simulink model "SpaceRendezvousAndDockingExample"  (R2025a)
settings: Solver=ode45  StartTime=0.0  StopTime=endTime  RelTol=1e-10  AbsTol=1e-10
PreLoadFcn:
  | % Variables to allow model to run without example script
  | primaryAlignmentVector = [1;0;0];
  | secondaryAlignmentVector = [0;0;1];
  | endTime = 100000;
  | epochYear = 2022;
  | epochMonth = 8;
  | epochDay = 6;
  | epochHour = 0;
  | epochMinute = 0;
  | epochSecond = 0;
  | initialApproachClosingRate = 0.3;
  | finalApproachClosingRate1 = 0.3;
  | finalApproachClosingRate2 = 0.03;
  | primaryConstraintVectorTarget = [1;0;0];
  | secondaryConstraintVectorTarget= [0;0;1];
  | collisionAvoidanceZOffset = 20;
  | transpositionFinalPosition = [20;0;0];
  | m0 = 1000;
  | mDot = 7500;
  | ve = 3924;
  | initialTargetSemimajorAxis = 8000000;
  | initialTargetEccentricity = 0.0005;
  | initialTargetInclination = 30;
  | initialTargetRightAscensionofAscendingNode = 60;
  | initialTargetArgumentOfPeriapsis = 120;
  | initialTargetTrueAnomaly = 310;
  | targetAttitude = [1 0 0 0];
  | initialChaserSemimajorAxis = 7500000;
  | initialChaserEccentricity = 0.001;
  | initialChaserInclination = 30.1;
  | initialChaserRightAscensionofAscendingNode = 60.1;
  | initialChaserArgumentOfPeriapsis = 120;
  | initialChaserTrueAnomaly = 30;
  | burnDirection1 = [-0.0281; 0.9382; 0.3450];
  | burnDirection2 = [-0.1134;-0.9766;-0.1829];
  | burnDuration1 = 0.0100;
  | burnDuration2 = 0.0049;
  | burnTime1 = 1430.892;
  | burnTime2 = 79222.205;
undefined symbols (not defined in the file or in its folder): juliandate
libraries: aerolibutil x12, aerolibsatdyn x2, simulink x2, matrix_library x1
CloseFcn:
  | clear primaryAlignmentVector secondaryAlignmentVector;
  | clear endTime epochYear epochMonth epochDay;
  | clear epochHour epochMinute epochSecond;
  | clear initialApproachClosingRate;
  | clear finalApproachClosingRate1 finalApproachClosingRate2;
  | clear primaryConstraintVectorTarget secondaryConstraintVectorTarget;
  | clear collisionAvoidanceZOffset transpositionFinalPosition;
  | clear m0 mDot ve;
  | clear initialTargetSemimajorAxis initialTargetRightAscensionofAscendingNode;
  | clear initialTargetArgumentOfPeriapsis initialTargetInclination initialTargetEccentricity;
  | clear initialTargetTrueAnomaly targetAttitude;
  | clear initialChaserSemimajorAxis initialChaserRightAscensionofAscendingNode;
  | clear initialChaserArgumentOfPeriapsis initialChaserInclination initialChaserEccentricity;
  | clear initialChaserTrueAnomaly;
  | clear burnDirection1 burnDirection2 burnDuration1 burnDuration2;
  | clear burnTime1 burnTime2;
settings Model: SimulationMode=accelerator  ExtModeTrigDuration=100  Creator=The MathWorks, Inc.  LastModifiedBy=aylin
settings SolverCC: ConsecutiveZCsStepRelTol=eps  ZeroCrossControl=EnableAll
settings DataIOCC: StateSaveName=tmp_raccel_xout  SignalLoggingName=tmp_raccel_logsout
settings OptimizationCC: ReuseModelBlockBuffer=off  EfficientMapNaN2IntZero=off
settings HardwareCC: TargetBitPerPointer=64.0  TargetBitPerSizeT=64.0  TargetBitPerPtrDiffT=64.0  TargetLongLongMode=on  TargetIntDivRoundTo=Zero  TargetEndianess=LittleEndian  TargetWordSize=64.0  TargetHWDeviceType=MATLAB Host  ProdEqTarget=off
settings RTWCC: SystemTargetFile=raccel.tlc  TemplateMakefile=raccel_default_tmf  RTWVerbose=off  RTWUseSimCustomCode=on  CustomBLASCallback=coder.internal.blas.MATLABBLASCallback  GPUComputeCapability=3.5
settings CodeAppCC: GenerateComments=off  MaxIdLength=128.0  MangleLength=10.0  SimulinkBlockComments=off
settings RaccelTargetCC: ExtModeTransport=0.0  ExtModeStaticAllocSize=1000000.0  ENABLE_SLEXEC_SSBRIDGE=1.0  RTWCAPIParams=on  RTWCAPIRootIO=on  TargetLangStandard=C99 (ISO)  MultiwordLength=2048.0  DynamicStringBufferSize=256.0  PreserveMATLABNamespacesInGeneratedCode=on  SubcomponentCodeInterfacePackaging=Reusable function  InstructionSetFMA=off  OptimizeReductions=off  LogToMDFFile=off

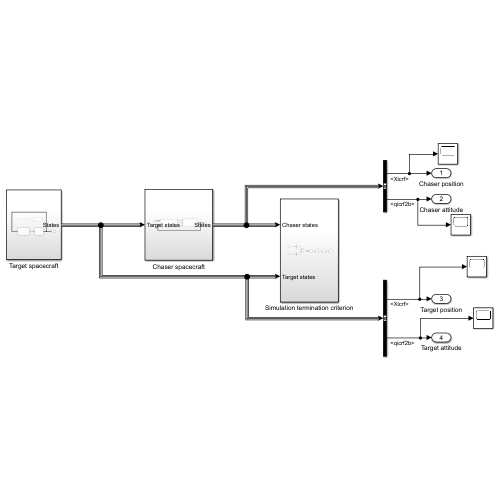
[thumbnail: Simulink's stored preview of the top-level diagram]
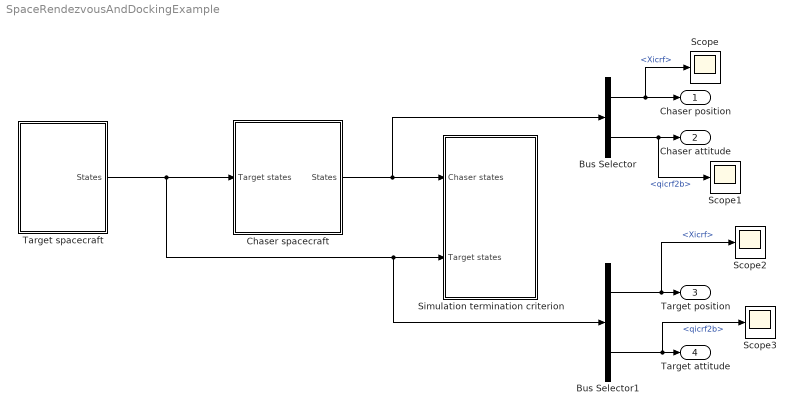
== system SpaceRendezvousAndDockingExample ==
  Bus Selector : BusSelector  OutputSignals=Xicrf,qicrf2b
  Bus Selector1 : BusSelector  OutputSignals=Xicrf,qicrf2b
  Chaser spacecraft : Subsystem
  Scope{,1..3} (4 alike) : Scope
      Scope settings: ActiveDisplayYMinimum=-9.6776650490296111E+6  ActiveDisplayYMaximum=9.6954640702499E+6
      Scope1 settings: ActiveDisplayYMinimum=-1.2116665545689753  ActiveDisplayYMaximum=1.2457407282854416
      Scope2 settings: ActiveDisplayYMinimum=-9.6822251081786063E+6  ActiveDisplayYMaximum=9.6826892101331856E+6  DataLoggingVariableName=ScopeData2
      Scope3 settings: ActiveDisplayYMinimum=-0.12500337803763709  ActiveDisplayYMaximum=1.1250003753375153  DataLoggingVariableName=ScopeData3
  Simulation termination criterion : Subsystem
  Target spacecraft : Subsystem
  Chaser position : Outport
  Chaser attitude : Outport  Port=2
  Target position : Outport  Port=3
  Target attitude : Outport  Port=4
  wires:
  Chaser spacecraft/1(States) -> Bus Selector/1, Simulation termination criterion/1(Chaser states)
  Target spacecraft/1(States) -> Chaser spacecraft/1(Target states), Bus Selector1/1, Simulation termination criterion/2(Target states)
  Bus Selector/1 -> Scope/1, Chaser position/1  "<Xicrf>"
  Bus Selector/2 -> Scope1/1, Chaser attitude/1  "<qicrf2b>"
  Bus Selector1/1 -> Scope2/1, Target position/1  "<Xicrf>"
  Bus Selector1/2 -> Scope3/1, Target attitude/1  "<qicrf2b>"

== system SpaceRendezvousAndDockingExample/Chaser spacecraft ==
  Target states : Inport
  Guidance and control : Subsystem  TreatAsAtomicUnit=on
  Spacecraft : Subsystem
  States : Outport
  wires:
  Target states/1 -> Guidance and control/1(Target states)
  Guidance and control/2(Fb) -> Spacecraft/2(Fb)
  Guidance and control/1(Main engine burn command) -> Spacecraft/1(Main engine burn command)
  Guidance and control/3(Mb) -> Spacecraft/3(Mb)
  Spacecraft/1(States) -> Guidance and control/2(States), States/1

== system SpaceRendezvousAndDockingExample/Simulation termination criterion ==
  Chaser states : Inport
  Target states : Inport  Port=2
  Bus Selector : BusSelector  OutputSignals=Xicrf
  Bus Selector1 : BusSelector  OutputSignals=Xicrf
  Compare To Constant : simulink/Logic and Bit Operations/Compare To Constant  relop=<=  const=1  OutDataTypeStr=boolean
  Dot Product : DotProduct  OutDataTypeStr=Inherit: Inherit via internal rule
  Sqrt : Sqrt
  Stop Simulation : Stop
  Sum : Sum  Inputs=+-
  wires:
  Sqrt/1 -> Compare To Constant/1
  Compare To Constant/1 -> Stop Simulation/1
  Sum/1 -> Dot Product/2, Dot Product/1
  Dot Product/1 -> Sqrt/1
  Target states/1 -> Bus Selector1/1
  Chaser states/1 -> Bus Selector/1
  Bus Selector/1 -> Sum/1  "<Xicrf>"
  Bus Selector1/1 -> Sum/2  "<Xicrf>"

== system SpaceRendezvousAndDockingExample/Target spacecraft ==
  Guidance and control : Subsystem  TreatAsAtomicUnit=on
  Sensors Dynamics : Subsystem  Commented=on
  Spacecraft : Subsystem
  States : Outport
  wires:
  Guidance and control/1(Mb) -> Spacecraft/1(Mb)
  Spacecraft/1(States) -> Guidance and control/1(States), States/1
  Sensors Dynamics/1(Out1) -> ?

== system SpaceRendezvousAndDockingExample/Chaser spacecraft/Guidance and control ==
  Target states : Inport
  States : Inport  Port=2
  Control : Subsystem  TreatAsAtomicUnit=on
  Guidance : Subsystem  TreatAsAtomicUnit=on
  Main engine burn command : Outport
  Fb : Outport  Port=2
  Mb : Outport  Port=3
  wires:
  Control/2(Mb) -> Mb/1
  Control/1(Fb) -> Fb/1
  States/1 -> Guidance/2(States), Control/5(States)
  Target states/1 -> Guidance/1(Target states), Control/4(Target states)
  Guidance/1(Main engine burn command) -> Main engine burn command/1
  Guidance/2(Translational guidance) -> Control/1(Translational guidance)
  Guidance/3(Rotational guidance) -> Control/2(Rotational guidance)
  Guidance/4(Enable translational control) -> Control/3(Enable translational control)

== system SpaceRendezvousAndDockingExample/Chaser spacecraft/Spacecraft ==
  Main engine burn command : Inport
  Fb : Inport  Port=2
  Mb : Inport  Port=3
  Bus Creator : BusCreator  Inputs=4
  Exhaust velocity : Constant  Value=[-ve;0;0]
  Max mass flow rate : Gain  Gain=-mDot
  Spacecraft Dynamics : SpacecraftDynamics  startDate=juliandate(epochYear,epochMonth,epochDay,epochHour,epochMinute,epochSecond)  dateOut=off  massType=Simple variable  mass=m0  emptyMass=300  fullMass=m0  emptyInertia=[250, 0, 0; 0, 336.75, 0; 0, 0,336.75]  fullInertia=[500, 0, 0; 0, 2500, 0; 0, 0,2500]  useMassFlowRelativeVelocity=on  outputFuelStatus=off  semiMajorAxis=initialChaserSemimajorAxis  eccentricity=initialChaserEccentricity  inclination=initialChaserInclination  raan=initialChaserRightAscensionofAscendingNode  argPeriapsis=initialChaserArgumentOfPeriapsis  trueAnomaly=initialChaserTrueAnomaly  inertialPosition=[0,-10000000,0]  inertialVelocity=[8000,0,0]  attitude=targetAttitude  attitudeRate=[0.01, 0.002, 0]  gravityModel=Point-mass  useDrag=on  useSRP=on
  States : Outport
  wires:
  Max mass flow rate/1 -> Spacecraft Dynamics/3
  Fb/1 -> Spacecraft Dynamics/1
  Exhaust velocity/1 -> Spacecraft Dynamics/4
  Mb/1 -> Spacecraft Dynamics/2
  Main engine burn command/1 -> Max mass flow rate/1
  Bus Creator/1 -> States/1
  Spacecraft Dynamics/4 -> Bus Creator/4  "wicrf2b"
  Spacecraft Dynamics/2 -> Bus Creator/2  "Vicrf"
  Spacecraft Dynamics/1 -> Bus Creator/1  "Xicrf"
  Spacecraft Dynamics/3 -> Bus Creator/3  "qicrf2b"

== system SpaceRendezvousAndDockingExample/Target spacecraft/Guidance and control ==
  States : Inport
  Rotational controller : Subsystem  TreatAsAtomicUnit=on  SystemSampleTime=1/10
  Rotational guidance : Subsystem  TreatAsAtomicUnit=on
  Mb : Outport
  wires:
  Rotational controller/1(Mb) -> Mb/1
  States/1 -> Rotational controller/2(States)
  Rotational guidance/1(Rotational guidance) -> Rotational controller/1(Rotational guidance)

== system SpaceRendezvousAndDockingExample/Target spacecraft/Sensors Dynamics ==
  In1 : Inport
  Add : Sum
  Band-Limited White Noise : simulink/Sources/Band-Limited White Noise  Cov=[0.1]  Ts=0.1  seed=[23341]
  Out1 : Outport
  wires:
  In1/1 -> Add/2
  Band-Limited White Noise/1 -> Add/1
  Add/1 -> Out1/1

== system SpaceRendezvousAndDockingExample/Target spacecraft/Spacecraft ==
  Mb : Inport
  Bus Creator : BusCreator  Inputs=4
  Spacecraft Dynamics : SpacecraftDynamics  forcesIn=off  startDate=juliandate(epochYear,epochMonth,epochDay,epochHour,epochMinute,epochSecond)  dateOut=off  mass=m0  emptyMass=300  fullMass=1000  inertia=[500, 0, 0; 0, 2500, 0; 0, 0,2500]  emptyInertia=[250, 0, 0; 0, 336.75, 0; 0, 0,336.75]  fullInertia=[500, 0, 0; 0, 2500, 0; 0, 0,2500]  outputFuelStatus=off  semiMajorAxis=initialTargetSemimajorAxis  eccentricity=initialTargetEccentricity  inclination=initialTargetInclination  raan=initialTargetRightAscensionofAscendingNode  argPeriapsis=initialTargetArgumentOfPeriapsis  trueAnomaly=initialTargetTrueAnomaly  inertialPosition=[0,-10000000,0]  inertialVelocity=[8000,0,0]  attitude=targetAttitude  attitudeRate=[0.005, 0.02, 0.01]  gravityModel=Point-mass  useDrag=on  useSRP=on
  States : Outport
  wires:
  Spacecraft Dynamics/1 -> Bus Creator/1  "Xicrf"
  Spacecraft Dynamics/4 -> Bus Creator/4  "wicrf2b"
  Bus Creator/1 -> States/1
  Spacecraft Dynamics/2 -> Bus Creator/2  "Vicrf"
  Spacecraft Dynamics/3 -> Bus Creator/3  "qicrf2b"
  Mb/1 -> Spacecraft Dynamics/1

== system SpaceRendezvousAndDockingExample/Chaser spacecraft/Guidance and control/Control ==
  Translational guidance : Inport
  Rotational guidance : Inport  Port=2
  Enable translational control : Inport  Port=3
  Target states : Inport  Port=4
  States : Inport  Port=5
  Rotational controller : Subsystem  TreatAsAtomicUnit=on  SystemSampleTime=1/10
  Translational controller : Subsystem  TreatAsAtomicUnit=on
  Fb : Outport
  Mb : Outport  Port=2
  wires:
  Enable translational control/1 -> Translational controller/Enable
  Rotational controller/2(Mb) -> Mb/1
  Translational controller/1(Fb) -> Fb/1
  Target states/1 -> Translational controller/1(Target states)
  States/1 -> Translational controller/2(States), Rotational controller/1(States)
  Translational guidance/1 -> Translational controller/3(Translation guidance)
  Rotational controller/1(Pointing complete) -> Translational controller/4(Pointing complete)
  Rotational guidance/1 -> Rotational controller/2(Rotational guidance)

== system SpaceRendezvousAndDockingExample/Chaser spacecraft/Guidance and control/Guidance ==
  Target states : Inport
  States : Inport  Port=2
  Clock : Clock
  Maneuver : Subsystem
  Maneuver selector : Stateflow chart  TreatAsAtomicUnit=on
  Main engine burn command : Outport
  Translational guidance : Outport  Port=2
  Rotational guidance : Outport  Port=3
  Enable translational control : Outport  Port=4
  wires:
  Clock/1 -> Maneuver selector/1(missionTime)
  Maneuver selector/3(enableDocking) -> Maneuver/3(Enable docking), Enable translational control/1
  Target states/1 -> Maneuver/4(Target states)
  States/1 -> Maneuver/5(States)
  Maneuver/1(Main engine burn command) -> Main engine burn command/1
  Maneuver/2(Translational guidance) -> Translational guidance/1
  Maneuver/3(Rotational guidance) -> Rotational guidance/1
  Maneuver selector/1(enableRendezvousManeuver1) -> Maneuver/1(Enable rendezvous maneuver 1)
  Maneuver selector/2(enableRendezvousManeuver2) -> Maneuver/2(Enable rendezvous maneuver 2)

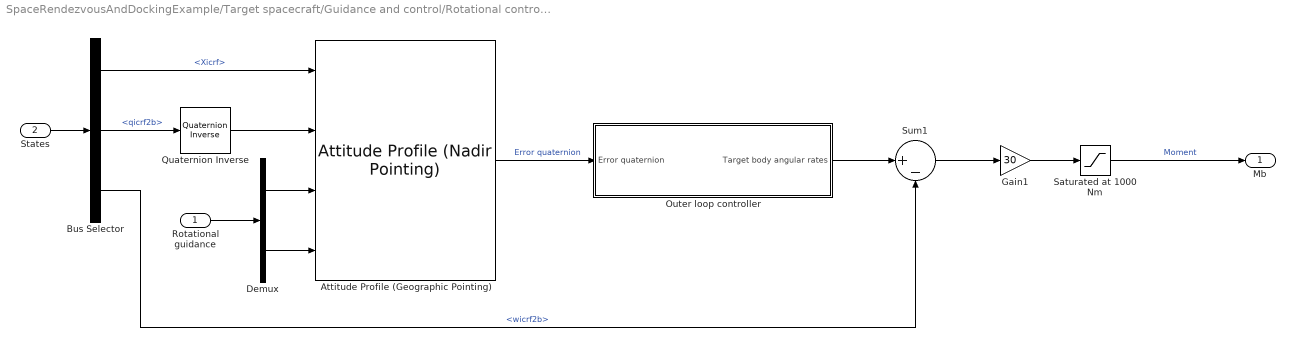
== system SpaceRendezvousAndDockingExample/Target spacecraft/Guidance and control/Rotational controller ==
  Rotational guidance : Inport
  States : Inport  Port=2
  Attitude Profile (Geographic Pointing) : aerolibsatdyn/Attitude Profile (Nadir Pointing)  outputError=on  outputFinalAttitude=off  portFrame=ICRF  pointingMode=Custom  celestialTarget=Sun  tunablePointing=off  primaryAlignmentSrc=Dialog  primaryAlignment=primaryAlignmentVector  secondaryAlignmentSrc=Dialog  secondaryAlignment=secondaryAlignmentVector  constraintFrame=ICRF  primaryConstraintSrc=Port  primaryConstraint=[1 0 0]  secondaryConstraintSrc=Port  secondaryConstraint=[0 0 1]
  Bus Selector : BusSelector  OutputSignals=Xicrf,qicrf2b,wicrf2b
  Demux : Demux  Outputs=2
  Gain1 : Gain  Gain=30
  Outer loop controller : Subsystem
  Quaternion Inverse : aerolibutil/Quaternion Inverse
  Saturated at 1000 Nm : Saturate  UpperLimit=1000  LowerLimit=-1000
  Sum1 : Sum  Inputs=|+-
  Mb : Outport
  wires:
  Gain1/1 -> Saturated at 1000 Nm/1
  Sum1/1 -> Gain1/1
  Quaternion Inverse/1 -> Attitude Profile (Geographic Pointing)/2
  Bus Selector/3 -> Sum1/2  "<wicrf2b>"
  States/1 -> Bus Selector/1
  Bus Selector/1 -> Attitude Profile (Geographic Pointing)/1  "<Xicrf>"
  Bus Selector/2 -> Quaternion Inverse/1  "<qicrf2b>"
  Rotational guidance/1 -> Demux/1
  Demux/2 -> Attitude Profile (Geographic Pointing)/4
  Demux/1 -> Attitude Profile (Geographic Pointing)/3
  Saturated at 1000 Nm/1 -> Mb/1  "Moment"
  Attitude Profile (Geographic Pointing)/1 -> Outer loop controller/1(Error quaternion)  "Error quaternion"
  Outer loop controller/1(Target body angular rates) -> Sum1/1

== system SpaceRendezvousAndDockingExample/Target spacecraft/Guidance and control/Rotational guidance ==
  Mux : Mux  Inputs=2
  Primary constraint vector : Constant  Value=primaryConstraintVectorTarget
  Secondary constraint vector : Constant  Value=secondaryConstraintVectorTarget
  Rotational guidance : Outport
  wires:
  Primary constraint vector/1 -> Mux/1
  Secondary constraint vector/1 -> Mux/2
  Mux/1 -> Rotational guidance/1

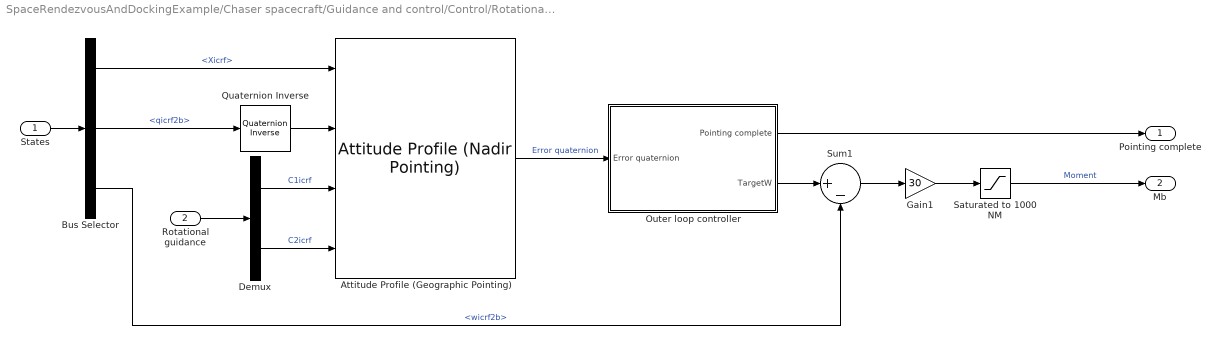
== system SpaceRendezvousAndDockingExample/Chaser spacecraft/Guidance and control/Control/Rotational controller ==
  States : Inport
  Rotational guidance : Inport  Port=2
  Attitude Profile (Geographic Pointing) : aerolibsatdyn/Attitude Profile (Nadir Pointing)  outputError=on  outputFinalAttitude=off  portFrame=ICRF  pointingMode=Custom  celestialTarget=Sun  tunablePointing=off  primaryAlignmentSrc=Dialog  primaryAlignment=primaryAlignmentVector  secondaryAlignmentSrc=Dialog  secondaryAlignment=secondaryAlignmentVector  constraintFrame=ICRF  primaryConstraintSrc=Port  primaryConstraint=[1 0 0]  secondaryConstraintSrc=Port  secondaryConstraint=[0 0 1]
  Bus Selector : BusSelector  OutputSignals=Xicrf,qicrf2b,wicrf2b
  Demux : Demux  Outputs=2
  Gain1 : Gain  Gain=30
  Outer loop controller : Subsystem
  Quaternion Inverse : aerolibutil/Quaternion Inverse
  Saturated to 1000 NM : Saturate  UpperLimit=1000  LowerLimit=-1000
  Sum1 : Sum  Inputs=|+-
  Pointing complete : Outport
  Mb : Outport  Port=2
  wires:
  Gain1/1 -> Saturated to 1000 NM/1
  Sum1/1 -> Gain1/1
  Bus Selector/2 -> Quaternion Inverse/1  "<qicrf2b>"
  States/1 -> Bus Selector/1
  Quaternion Inverse/1 -> Attitude Profile (Geographic Pointing)/2
  Bus Selector/3 -> Sum1/2  "<wicrf2b>"
  Bus Selector/1 -> Attitude Profile (Geographic Pointing)/1  "<Xicrf>"
  Rotational guidance/1 -> Demux/1
  Demux/1 -> Attitude Profile (Geographic Pointing)/3  "C1icrf"
  Demux/2 -> Attitude Profile (Geographic Pointing)/4  "C2icrf"
  Saturated to 1000 NM/1 -> Mb/1  "Moment"
  Attitude Profile (Geographic Pointing)/1 -> Outer loop controller/1(Error quaternion)  "Error quaternion"
  Outer loop controller/1(Pointing complete) -> Pointing complete/1
  Outer loop controller/2(TargetW) -> Sum1/1

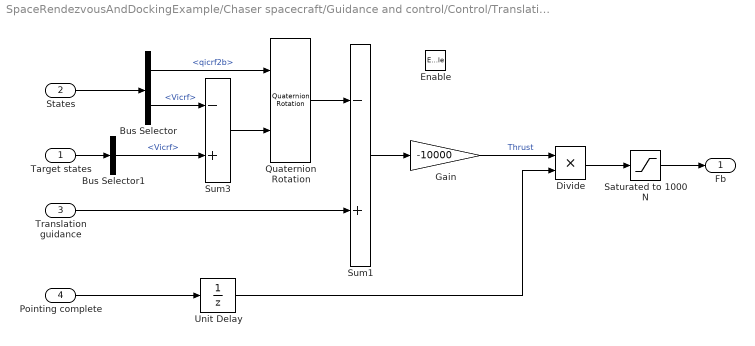
== system SpaceRendezvousAndDockingExample/Chaser spacecraft/Guidance and control/Control/Translational controller ==
  Target states : Inport
  States : Inport  Port=2
  Translation guidance : Inport  Port=3
  Pointing complete : Inport  Port=4
  Enable : EnablePort
  Bus Selector : BusSelector  OutputSignals=qicrf2b,Vicrf
  Bus Selector1 : BusSelector  OutputSignals=Vicrf
  Divide : Product  Inputs=**
  Gain : Gain  Gain=-10000
  Quaternion Rotation : aerolibutil/Quaternion Rotation
  Saturated to 1000 N : Saturate  UpperLimit=1000  LowerLimit=-1000
  Sum1 : Sum  Inputs=-+
  Sum3 : Sum  Inputs=-+
  Unit Delay : UnitDelay  InitialCondition=1  SampleTime=-1  HasFrameUpgradeWarning=on
  Fb : Outport  OutputWhenDisabled=reset  InitialOutput=[0 0 0]
  wires:
  States/1 -> Bus Selector/1
  Quaternion Rotation/1 -> Sum1/1
  Bus Selector/2 -> Sum3/1  "<Vicrf>"
  Sum3/1 -> Quaternion Rotation/2
  Translation guidance/1 -> Sum1/2
  Sum1/1 -> Gain/1
  Gain/1 -> Divide/1  "Thrust"
  Divide/1 -> Saturated to 1000 N/1
  Pointing complete/1 -> Unit Delay/1
  Saturated to 1000 N/1 -> Fb/1
  Unit Delay/1 -> Divide/2
  Bus Selector/1 -> Quaternion Rotation/1  "<qicrf2b>"
  Target states/1 -> Bus Selector1/1
  Bus Selector1/1 -> Sum3/2  "<Vicrf>"

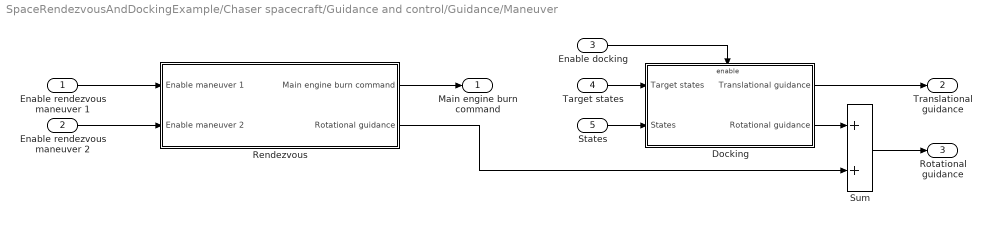
== system SpaceRendezvousAndDockingExample/Chaser spacecraft/Guidance and control/Guidance/Maneuver ==
  Enable rendezvous maneuver 1 : Inport
  Enable rendezvous maneuver 2 : Inport  Port=2
  Enable docking : Inport  Port=3
  Target states : Inport  Port=4
  States : Inport  Port=5
  Docking : Subsystem
  Rendezvous : Subsystem
  Sum : Sum
  Main engine burn command : Outport
  Translational guidance : Outport  Port=2
  Rotational guidance : Outport  Port=3
  wires:
  Target states/1 -> Docking/1(Target states)
  States/1 -> Docking/2(States)
  Enable docking/1 -> Docking/Enable
  Docking/1(Translational guidance) -> Translational guidance/1
  Docking/2(Rotational guidance) -> Sum/1
  Sum/1 -> Rotational guidance/1
  Enable rendezvous maneuver 1/1 -> Rendezvous/1(Enable maneuver 1)
  Enable rendezvous maneuver 2/1 -> Rendezvous/2(Enable maneuver 2)
  Rendezvous/2(Rotational guidance) -> Sum/2
  Rendezvous/1(Main engine burn command) -> Main engine burn command/1

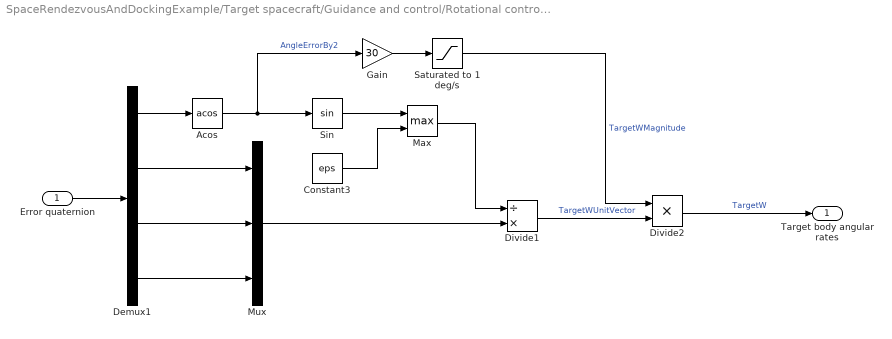
== system SpaceRendezvousAndDockingExample/Target spacecraft/Guidance and control/Rotational controller/Outer loop controller ==
  Error quaternion : Inport
  Acos : Trigonometry  Operator=acos
  Constant3 : Constant  Value=eps
  Demux1 : Demux
  Divide1 : Product  Inputs=/*
  Divide2 : Product  Inputs=**
  Gain : Gain  Gain=30
  Max : MinMax  Function=max  Inputs=2
  Mux : Mux  Inputs=3
  Saturated to 1 deg/s : Saturate  UpperLimit=1  LowerLimit=-1
  Sin : Trigonometry
  Target body angular rates : Outport
  wires:
  Mux/1 -> Divide1/2
  Demux1/2 -> Mux/1
  Saturated to 1 deg/s/1 -> Divide2/1  "TargetWMagnitude"
  Sin/1 -> Max/1
  Acos/1 -> Sin/1, Gain/1  "AngleErrorBy2"
  Divide1/1 -> Divide2/2  "TargetWUnitVector"
  Demux1/4 -> Mux/3
  Demux1/3 -> Mux/2
  Max/1 -> Divide1/1
  Demux1/1 -> Acos/1
  Constant3/1 -> Max/2
  Gain/1 -> Saturated to 1 deg/s/1
  Divide2/1 -> Target body angular rates/1  "TargetW"
  Error quaternion/1 -> Demux1/1

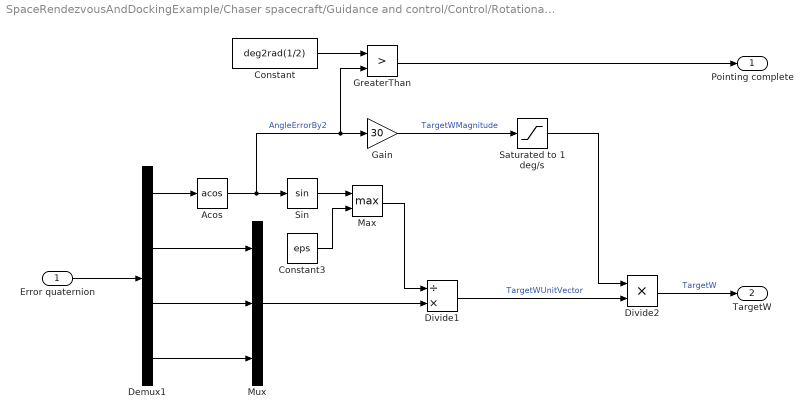
== system SpaceRendezvousAndDockingExample/Chaser spacecraft/Guidance and control/Control/Rotational controller/Outer loop controller ==
  Error quaternion : Inport
  Acos : Trigonometry  Operator=acos
  Constant : Constant  Value=deg2rad(1/2)
  Constant3 : Constant  Value=eps
  Demux1 : Demux
  Divide1 : Product  Inputs=/*
  Divide2 : Product  Inputs=**
  Gain : Gain  Gain=30
  GreaterThan : RelationalOperator  Operator=>  OutDataTypeStr=boolean  RndMeth=Simplest  InputSameDT=off
  Max : MinMax  Function=max  Inputs=2
  Mux : Mux  Inputs=3
  Saturated to 1 deg/s : Saturate  UpperLimit=1  LowerLimit=-1
  Sin : Trigonometry
  Pointing complete : Outport
  TargetW : Outport  Port=2
  wires:
  Divide1/1 -> Divide2/2  "TargetWUnitVector"
  Constant/1 -> GreaterThan/1
  Constant3/1 -> Max/2
  Mux/1 -> Divide1/2
  Acos/1 -> Sin/1, Gain/1, GreaterThan/2  "AngleErrorBy2"
  Sin/1 -> Max/1
  Demux1/3 -> Mux/2
  Demux1/1 -> Acos/1
  Gain/1 -> Saturated to 1 deg/s/1  "TargetWMagnitude"
  Divide2/1 -> TargetW/1  "TargetW"
  Demux1/4 -> Mux/3
  Demux1/2 -> Mux/1
  Max/1 -> Divide1/1
  Saturated to 1 deg/s/1 -> Divide2/1
  Error quaternion/1 -> Demux1/1
  GreaterThan/1 -> Pointing complete/1

== system SpaceRendezvousAndDockingExample/Chaser spacecraft/Guidance and control/Guidance/Maneuver/Docking ==
  Target states : Inport
  States : Inport  Port=2
  Enable : EnablePort
  Docking phase guidance : Subsystem
  Docking phase selector : Subsystem
  Translational guidance : Outport  OutputWhenDisabled=reset  InitialOutput=[0 0 0]
  Rotational guidance : Outport  Port=2  OutputWhenDisabled=reset  InitialOutput=[0 0 0 0 0 0]
  wires:
  Target states/1 -> Docking phase selector/2(Target states), Docking phase guidance/4(Target states)
  States/1 -> Docking phase selector/3(States), Docking phase guidance/5(States)
  Docking phase guidance/2(Translation guidance) -> Translational guidance/1
  Docking phase guidance/1(transpositionError) -> Docking phase selector/1(Transposition error)
  Docking phase selector/1(Enable proximity ops) -> Docking phase guidance/1(Enable proximity ops)
  Docking phase selector/2(Enable transposition) -> Docking phase guidance/2(Enable transposition)
  Docking phase selector/3(Enable final approach) -> Docking phase guidance/3(Enable final approach)
  Docking phase guidance/3(Rotational guidance) -> Rotational guidance/1

== system SpaceRendezvousAndDockingExample/Chaser spacecraft/Guidance and control/Guidance/Maneuver/Rendezvous ==
  Enable maneuver 1 : Inport
  Enable maneuver 2 : Inport  Port=2
  Maneuver 1 : Subsystem
  Maneuver 2 : Subsystem
  Sum : Sum  Inputs=++|
  Sum1 : Sum  Inputs=|++
  Main engine burn command : Outport
  Rotational guidance : Outport  Port=2
  wires:
  Enable maneuver 1/1 -> Maneuver 1/Enable
  Enable maneuver 2/1 -> Maneuver 2/Enable
  Maneuver 2/2(Rotational guidance) -> Sum1/1
  Maneuver 1/2(Rotational guidance) -> Sum1/2
  Maneuver 2/1(Main engine burn command) -> Sum/2
  Maneuver 1/1(Main engine burn command) -> Sum/1
  Sum/1 -> Main engine burn command/1
  Sum1/1 -> Rotational guidance/1

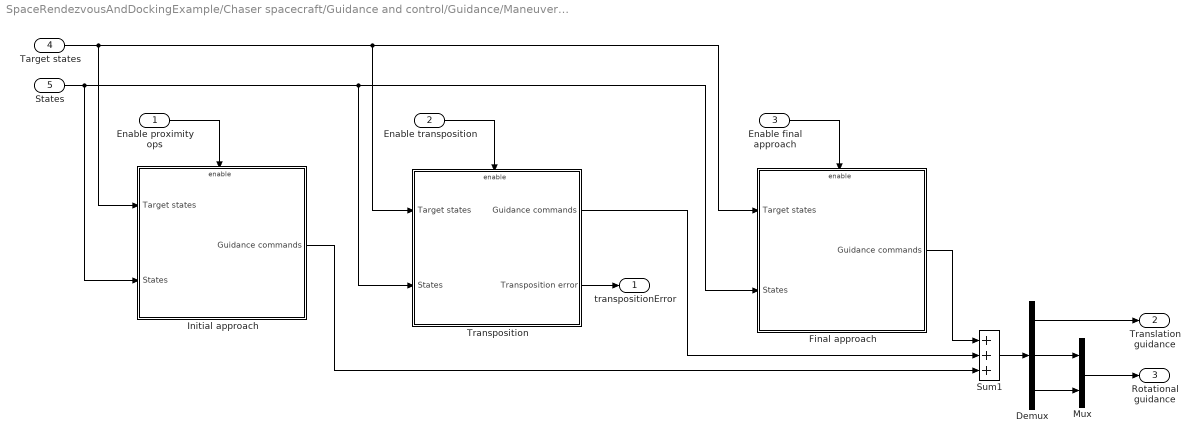
== system SpaceRendezvousAndDockingExample/Chaser spacecraft/Guidance and control/Guidance/Maneuver/Docking/Docking phase guidance ==
  Enable proximity ops : Inport
  Enable transposition : Inport  Port=2
  Enable final approach : Inport  Port=3
  Target states : Inport  Port=4
  States : Inport  Port=5
  Demux : Demux  Outputs=3
  Final approach : Subsystem
  Initial approach : Subsystem
  Mux : Mux  Inputs=2
  Sum1 : Sum  Inputs=+++
  Transposition : Subsystem
  transpositionError : Outport
  Translation guidance : Outport  Port=2
  Rotational guidance : Outport  Port=3
  wires:
  Enable proximity ops/1 -> Initial approach/Enable
  Sum1/1 -> Demux/1
  Enable transposition/1 -> Transposition/Enable
  Enable final approach/1 -> Final approach/Enable
  Target states/1 -> Transposition/1(Target states), Final approach/1(Target states), Initial approach/1(Target states)
  States/1 -> Initial approach/2(States), Final approach/2(States), Transposition/2(States)
  Final approach/1(Guidance commands) -> Sum1/1
  Transposition/1(Guidance commands) -> Sum1/2
  Initial approach/1(Guidance commands) -> Sum1/3
  Transposition/2(Transposition error) -> transpositionError/1
  Demux/1 -> Translation guidance/1
  Demux/2 -> Mux/1
  Demux/3 -> Mux/2
  Mux/1 -> Rotational guidance/1

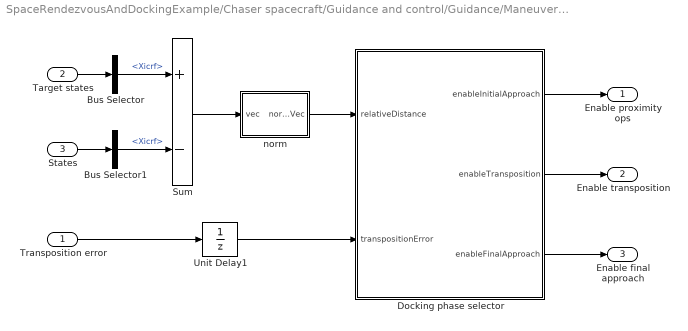
== system SpaceRendezvousAndDockingExample/Chaser spacecraft/Guidance and control/Guidance/Maneuver/Docking/Docking phase selector ==
  Transposition error : Inport
  Target states : Inport  Port=2
  States : Inport  Port=3
  Bus Selector : BusSelector  OutputSignals=Xicrf
  Bus Selector1 : BusSelector  OutputSignals=Xicrf
  Docking phase selector : Stateflow chart  TreatAsAtomicUnit=on
  Sum : Sum  Inputs=+-
  Unit Delay1 : UnitDelay  SampleTime=-1  HasFrameUpgradeWarning=on
  norm : Subsystem
  Enable proximity ops : Outport
  Enable transposition : Outport  Port=2
  Enable final approach : Outport  Port=3
  wires:
  Unit Delay1/1 -> Docking phase selector/2(transpositionError)
  Target states/1 -> Bus Selector/1
  Sum/1 -> norm/1(vec)
  Docking phase selector/1(enableInitialApproach) -> Enable proximity ops/1
  norm/1(normVec) -> Docking phase selector/1(relativeDistance)
  Transposition error/1 -> Unit Delay1/1
  Docking phase selector/2(enableTransposition) -> Enable transposition/1
  Bus Selector/1 -> Sum/1  "<Xicrf>"
  States/1 -> Bus Selector1/1
  Bus Selector1/1 -> Sum/2  "<Xicrf>"
  Docking phase selector/3(enableFinalApproach) -> Enable final approach/1

== system SpaceRendezvousAndDockingExample/Chaser spacecraft/Guidance and control/Guidance/Maneuver/Rendezvous/Maneuver 1 ==
  Enable : EnablePort
  Constant : Constant  Value=burnDirection1
  Constant1 : Constant  Value=secondaryConstraintVectorTarget
  Mux : Mux  Inputs=2
  Off time = burnTime1 + burnDuration1 : Step  Time=burnTime1 + burnDuration1  SampleTime=0
  On time = burnTime1 : Step  Time=burnTime1  SampleTime=0
  Subtract : Sum  Inputs=+-
  Main engine burn command : Outport  OutputWhenDisabled=reset  InitialOutput=0
  Rotational guidance : Outport  Port=2  OutputWhenDisabled=reset  InitialOutput=[0 0 0 0 0 0]
  wires:
  Off time = burnTime1 + burnDuration1/1 -> Subtract/2
  On time = burnTime1/1 -> Subtract/1
  Subtract/1 -> Main engine burn command/1
  Constant/1 -> Mux/1
  Constant1/1 -> Mux/2
  Mux/1 -> Rotational guidance/1

== system SpaceRendezvousAndDockingExample/Chaser spacecraft/Guidance and control/Guidance/Maneuver/Rendezvous/Maneuver 2 ==
  Enable : EnablePort
  Constant : Constant  Value=burnDirection2
  Constant1 : Constant  Value=secondaryConstraintVectorTarget
  Mux : Mux  Inputs=2
  Off time = burnTime2 + burnDuration2 : Step  Time=burnTime2 + burnDuration2  SampleTime=0
  On time = burnTime2 : Step  Time=burnTime2  SampleTime=0
  Subtract1 : Sum  Inputs=+-
  Main engine burn command : Outport  OutputWhenDisabled=reset  InitialOutput=0
  Rotational guidance : Outport  Port=2  OutputWhenDisabled=reset  InitialOutput=[0 0 0 0 0 0]
  wires:
  On time = burnTime2/1 -> Subtract1/1
  Subtract1/1 -> Main engine burn command/1
  Constant/1 -> Mux/1
  Constant1/1 -> Mux/2
  Off time = burnTime2 + burnDuration2/1 -> Subtract1/2
  Mux/1 -> Rotational guidance/1

== system SpaceRendezvousAndDockingExample/Chaser spacecraft/Guidance and control/Guidance/Maneuver/Docking/Docking phase guidance/Final approach ==
  Target states : Inport
  States : Inport  Port=2
  Enable : EnablePort
  Mux : Mux  Inputs=3
  Rotational guidance : Subsystem
  Translational guidance : Subsystem  SystemSampleTime=0.1
  Guidance commands : Outport  OutputWhenDisabled=reset  InitialOutput=[0 0 0 0 0 0 0 0 0]
  wires:
  Translational guidance/1(Target relative velocity command) -> Mux/1
  States/1 -> Translational guidance/2(States)
  Rotational guidance/1(C1icrf) -> Mux/2
  Rotational guidance/2(C2icrf) -> Mux/3
  Target states/1 -> Rotational guidance/1(Target states), Translational guidance/1(Target states)
  Mux/1 -> Guidance commands/1

== system SpaceRendezvousAndDockingExample/Chaser spacecraft/Guidance and control/Guidance/Maneuver/Docking/Docking phase guidance/Initial approach ==
  Target states : Inport
  States : Inport  Port=2
  Enable : EnablePort
  Mux : Mux  Inputs=3
  Rotational guidance : Subsystem
  Translational guidance : Subsystem  SystemSampleTime=0.1
  Guidance commands : Outport  OutputWhenDisabled=reset  InitialOutput=[0 0 0 0 0 0 0 0 0]
  wires:
  Translational guidance/1(Target relative velocity command) -> Mux/1
  Rotational guidance/1(C1icrf) -> Mux/2
  Target states/1 -> Rotational guidance/1(Target states), Translational guidance/1(Target states)
  States/1 -> Translational guidance/2(States)
  Mux/1 -> Guidance commands/1
  Rotational guidance/2(C2icrf) -> Mux/3

== system SpaceRendezvousAndDockingExample/Chaser spacecraft/Guidance and control/Guidance/Maneuver/Docking/Docking phase guidance/Transposition ==
  Target states : Inport
  States : Inport  Port=2
  Enable : EnablePort
  Mux : Mux  Inputs=3
  Rotational guidance : Subsystem
  Translational guidance : Subsystem  SystemSampleTime=0.1
  Guidance commands : Outport  OutputWhenDisabled=reset  InitialOutput=[0 0 0 0 0 0 0 0 0]
  Transposition error : Outport  Port=2  OutputWhenDisabled=reset  InitialOutput=1
  wires:
  States/1 -> Translational guidance/2(States)
  Rotational guidance/1(C1icrf) -> Mux/2
  Rotational guidance/2(C2icrf) -> Mux/3
  Target states/1 -> Rotational guidance/1(Target states), Translational guidance/1(Target states)
  Translational guidance/2(Transposition error) -> Transposition error/1
  Mux/1 -> Guidance commands/1
  Translational guidance/1(Target relative velocity command) -> Mux/1

== system SpaceRendezvousAndDockingExample/Chaser spacecraft/Guidance and control/Guidance/Maneuver/Docking/Docking phase selector/norm ==
  vec : Inport
  Dot Product : DotProduct  OutDataTypeStr=Inherit: Inherit via internal rule
  Sqrt : Sqrt
  normVec : Outport
  wires:
  vec/1 -> Dot Product/2, Dot Product/1
  Dot Product/1 -> Sqrt/1
  Sqrt/1 -> normVec/1

== system SpaceRendezvousAndDockingExample/Chaser spacecraft/Guidance and control/Guidance/Maneuver/Docking/Docking phase guidance/Final approach/Rotational guidance ==
  Target states : Inport
  Bus Selector : BusSelector  OutputSignals=qicrf2b
  Constant : Constant  Value=[-1 0 0]
  Constant1 : Constant  Value=[0 0 1]
  Quaternion Inverse : aerolibutil/Quaternion Inverse
  Quaternion Rotation : aerolibutil/Quaternion Rotation
  Quaternion Rotation1 : aerolibutil/Quaternion Rotation
  C1icrf : Outport
  C2icrf : Outport  Port=2
  wires:
  Constant/1 -> Quaternion Rotation/2
  Constant1/1 -> Quaternion Rotation1/2
  Quaternion Rotation/1 -> C1icrf/1  "targetBodyFrameNegativeXAxis"
  Quaternion Rotation1/1 -> C2icrf/1  "targetBodyFrameZAxis"
  Target states/1 -> Bus Selector/1
  Quaternion Inverse/1 -> Quaternion Rotation1/1, Quaternion Rotation/1
  Bus Selector/1 -> Quaternion Inverse/1  "<qicrf2b>"

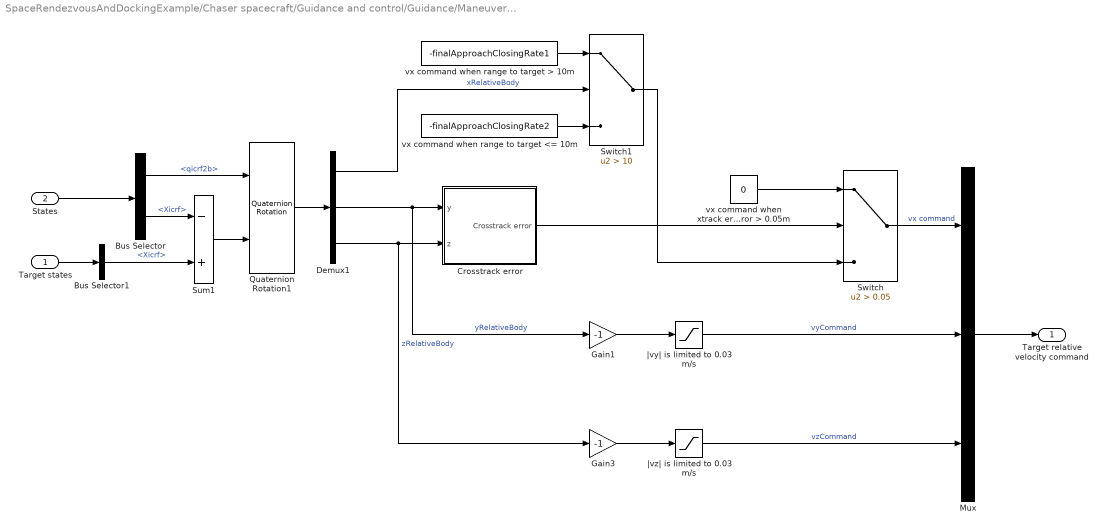
== system SpaceRendezvousAndDockingExample/Chaser spacecraft/Guidance and control/Guidance/Maneuver/Docking/Docking phase guidance/Final approach/Translational guidance ==
  Target states : Inport
  States : Inport  Port=2
  Bus Selector : BusSelector  OutputSignals=qicrf2b,Xicrf
  Bus Selector1 : BusSelector  OutputSignals=Xicrf
  Crosstrack error : Subsystem
  Demux1 : Demux  Outputs=3
  Gain1 : Gain  Gain=-1
  Gain3 : Gain  Gain=-1
  Mux : Mux  Inputs=3
  Quaternion Rotation1 : aerolibutil/Quaternion Rotation
  Sum1 : Sum  Inputs=-+
  Switch : Switch  Criteria=u2 > Threshold  Threshold=0.05  SaturateOnIntegerOverflow=off  InputSameDT=off
  Switch1 : Switch  Criteria=u2 > Threshold  Threshold=10  SaturateOnIntegerOverflow=off  InputSameDT=off
  vx command when range to target <= 10m : Constant  Value=-finalApproachClosingRate2
  vx command when range to target > 10m : Constant  Value=-finalApproachClosingRate1
  vx command when xtrack error > 0.05m : Constant  Value=0
  |vy| is limited to 0.03 m/s : Saturate  UpperLimit=0.03  LowerLimit=-0.03
  |vz| is limited to 0.03 m/s : Saturate  UpperLimit=0.03  LowerLimit=-0.03
  Target relative velocity command : Outport
  wires:
  Sum1/1 -> Quaternion Rotation1/2
  Quaternion Rotation1/1 -> Demux1/1
  Crosstrack error/1(Crosstrack error) -> Switch/2
  Switch1/1 -> Switch/3
  Demux1/1 -> Switch1/2  "xRelativeBody"
  Switch/1 -> Mux/1  "vx command"
  vx command when xtrack error > 0.05m/1 -> Switch/1
  Gain1/1 -> |vy| is limited to 0.03 m/s/1
  Gain3/1 -> |vz| is limited to 0.03 m/s/1
  |vz| is limited to 0.03 m/s/1 -> Mux/3  "vzCommand"
  |vy| is limited to 0.03 m/s/1 -> Mux/2  "vyCommand"
  Demux1/2 -> Gain1/1, Crosstrack error/1(y)  "yRelativeBody"
  Demux1/3 -> Gain3/1, Crosstrack error/2(z)  "zRelativeBody"
  Mux/1 -> Target relative velocity command/1
  vx command when range to target > 10m/1 -> Switch1/1
  vx command when range to target <= 10m/1 -> Switch1/3
  States/1 -> Bus Selector/1
  Bus Selector/1 -> Quaternion Rotation1/1  "<qicrf2b>"
  Bus Selector/2 -> Sum1/1  "<Xicrf>"
  Target states/1 -> Bus Selector1/1
  Bus Selector1/1 -> Sum1/2  "<Xicrf>"

== system SpaceRendezvousAndDockingExample/Chaser spacecraft/Guidance and control/Guidance/Maneuver/Docking/Docking phase guidance/Initial approach/Rotational guidance ==
  Target states : Inport
  Bus Selector : BusSelector  OutputSignals=Xicrf,Vicrf
  Cross Product : matrix_library/Cross Product
  Divide : Product  Inputs=*/
  Divide1 : Product  Inputs=*/
  Dot Product : DotProduct  OutDataTypeStr=Inherit: Inherit via internal rule
  Dot Product1 : DotProduct  OutDataTypeStr=Inherit: Inherit via internal rule
  Sqrt : Sqrt
  Sqrt1 : Sqrt
  C1icrf : Outport
  C2icrf : Outport  Port=2
  wires:
  Dot Product1/1 -> Sqrt1/1
  Sqrt1/1 -> Divide1/2
  Cross Product/1 -> Dot Product/2, Divide/1, Dot Product/1
  Bus Selector/1 -> Cross Product/1, Dot Product1/2, Divide1/1, Dot Product1/1  "<Xicrf>"
  Dot Product/1 -> Sqrt/1
  Sqrt/1 -> Divide/2
  Divide/1 -> C2icrf/1  "targetOrbitalAngularMomentumUnitVector"
  Divide1/1 -> C1icrf/1  "targetPositionUnitVector"
  Bus Selector/2 -> Cross Product/2  "<Vicrf>"
  Target states/1 -> Bus Selector/1

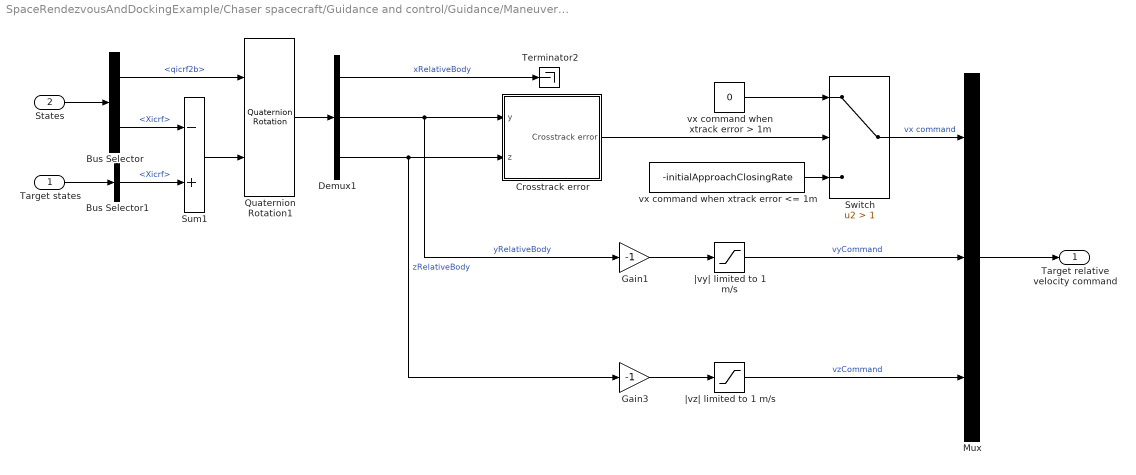
== system SpaceRendezvousAndDockingExample/Chaser spacecraft/Guidance and control/Guidance/Maneuver/Docking/Docking phase guidance/Initial approach/Translational guidance ==
  Target states : Inport
  States : Inport  Port=2
  Bus Selector : BusSelector  OutputSignals=qicrf2b,Xicrf
  Bus Selector1 : BusSelector  OutputSignals=Xicrf
  Crosstrack error : Subsystem
  Demux1 : Demux  Outputs=3
  Gain1 : Gain  Gain=-1
  Gain3 : Gain  Gain=-1
  Mux : Mux  Inputs=3
  Quaternion Rotation1 : aerolibutil/Quaternion Rotation
  Sum1 : Sum  Inputs=-+
  Switch : Switch  Criteria=u2 > Threshold  Threshold=1  SaturateOnIntegerOverflow=off  InputSameDT=off
  Terminator2 : Terminator
  vx command when xtrack error <= 1m : Constant  Value=-initialApproachClosingRate
  vx command when xtrack error > 1m : Constant  Value=0
  |vy| limited to 1 m/s : Saturate  UpperLimit=1  LowerLimit=-1
  |vz| limited to 1 m/s : Saturate  UpperLimit=1  LowerLimit=-1
  Target relative velocity command : Outport
  wires:
  Target states/1 -> Bus Selector1/1
  Sum1/1 -> Quaternion Rotation1/2
  Bus Selector/2 -> Sum1/1  "<Xicrf>"
  Bus Selector/1 -> Quaternion Rotation1/1  "<qicrf2b>"
  Quaternion Rotation1/1 -> Demux1/1
  Crosstrack error/1(Crosstrack error) -> Switch/2
  vx command when xtrack error <= 1m/1 -> Switch/3
  Demux1/1 -> Terminator2/1  "xRelativeBody"
  Switch/1 -> Mux/1  "vx command"
  vx command when xtrack error > 1m/1 -> Switch/1
  Gain1/1 -> |vy| limited to 1 m/s/1
  Gain3/1 -> |vz| limited to 1 m/s/1
  |vz| limited to 1 m/s/1 -> Mux/3  "vzCommand"
  |vy| limited to 1 m/s/1 -> Mux/2  "vyCommand"
  Demux1/2 -> Gain1/1, Crosstrack error/1(y)  "yRelativeBody"
  Demux1/3 -> Gain3/1, Crosstrack error/2(z)  "zRelativeBody"
  Mux/1 -> Target relative velocity command/1
  States/1 -> Bus Selector/1
  Bus Selector1/1 -> Sum1/2  "<Xicrf>"

== system SpaceRendezvousAndDockingExample/Chaser spacecraft/Guidance and control/Guidance/Maneuver/Docking/Docking phase guidance/Transposition/Rotational guidance ==
  Target states : Inport
  Bus Selector : BusSelector  OutputSignals=qicrf2b
  Constant : Constant  Value=[-1 0 0]
  Constant1 : Constant  Value=[0 0 1]
  Quaternion Inverse : aerolibutil/Quaternion Inverse
  Quaternion Rotation : aerolibutil/Quaternion Rotation
  Quaternion Rotation1 : aerolibutil/Quaternion Rotation
  C1icrf : Outport
  C2icrf : Outport  Port=2
  wires:
  Constant/1 -> Quaternion Rotation/2
  Constant1/1 -> Quaternion Rotation1/2
  Quaternion Rotation/1 -> C1icrf/1  "targetBodyFrameNegativeXAxis"
  Quaternion Rotation1/1 -> C2icrf/1  "targetBodyFrameZAxis"
  Target states/1 -> Bus Selector/1
  Quaternion Inverse/1 -> Quaternion Rotation1/1, Quaternion Rotation/1
  Bus Selector/1 -> Quaternion Inverse/1  "<qicrf2b>"

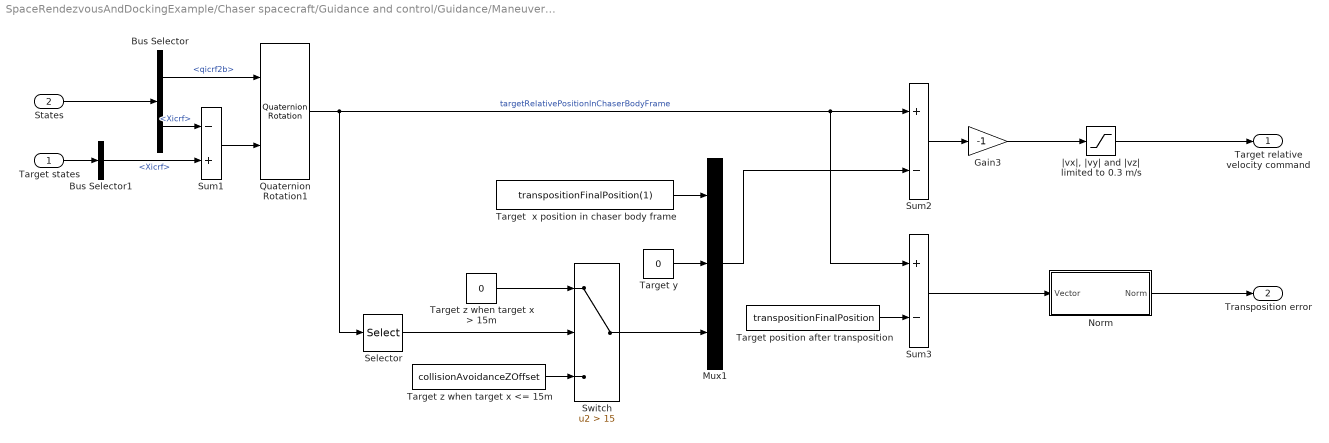
== system SpaceRendezvousAndDockingExample/Chaser spacecraft/Guidance and control/Guidance/Maneuver/Docking/Docking phase guidance/Transposition/Translational guidance ==
  Target states : Inport
  States : Inport  Port=2
  Bus Selector : BusSelector  OutputSignals=qicrf2b,Xicrf
  Bus Selector1 : BusSelector  OutputSignals=Xicrf
  Gain3 : Gain  Gain=-1
  Mux1 : Mux  Inputs=3
  Norm : Subsystem
  Quaternion Rotation1 : aerolibutil/Quaternion Rotation
  Selector : Selector  InputPortWidth=3  IndexOptions=Index vector (dialog)  Indices=[1]  OutputSizes=1
  Sum1 : Sum  Inputs=-+
  Sum2 : Sum  Inputs=+-
  Sum3 : Sum  Inputs=+-
  Switch : Switch  Criteria=u2 > Threshold  Threshold=15  SaturateOnIntegerOverflow=off  InputSameDT=off
  Target  x position in chaser body frame : Constant  Value=transpositionFinalPosition(1)
  Target position after transposition : Constant  Value=transpositionFinalPosition
  Target y : Constant  Value=0
  Target z when target x <= 15m : Constant  Value=collisionAvoidanceZOffset
  "Target z when target x > 15m " : Constant  Value=0
  "|vx|, |vy| and |vz| limited to 0.3 m/s" : Saturate  UpperLimit=0.3  LowerLimit=-0.3
  Target relative velocity command : Outport
  Transposition error : Outport  Port=2
  wires:
  Sum1/1 -> Quaternion Rotation1/2
  Quaternion Rotation1/1 -> Selector/1, Sum2/1, Sum3/1  "targetRelativePositionInChaserBodyFrame"
  "|vx|, |vy| and |vz| limited to 0.3 m/s"/1 -> Target relative velocity command/1
  Sum2/1 -> Gain3/1
  Gain3/1 -> "|vx|, |vy| and |vz| limited to 0.3 m/s"/1
  Norm/1(Norm) -> Transposition error/1
  States/1 -> Bus Selector/1
  Bus Selector/1 -> Quaternion Rotation1/1  "<qicrf2b>"
  Bus Selector/2 -> Sum1/1  "<Xicrf>"
  Target states/1 -> Bus Selector1/1
  Bus Selector1/1 -> Sum1/2  "<Xicrf>"
  "Target z when target x > 15m "/1 -> Switch/1
  Target z when target x <= 15m/1 -> Switch/3
  Target  x position in chaser body frame/1 -> Mux1/1
  Switch/1 -> Mux1/3
  Selector/1 -> Switch/2
  Mux1/1 -> Sum2/2
  Sum3/1 -> Norm/1(Vector)
  Target position after transposition/1 -> Sum3/2
  Target y/1 -> Mux1/2

== system SpaceRendezvousAndDockingExample/Chaser spacecraft/Guidance and control/Guidance/Maneuver/Docking/Docking phase guidance/Final approach/Translational guidance/Crosstrack error ==
  y : Inport
  z : Inport  Port=2
  Sqrt : Sqrt
  Square : Math  Operator=square
  Square1 : Math  Operator=square
  Sum : Sum
  Crosstrack error : Outport
  wires:
  z/1 -> Square1/1
  Sum/1 -> Sqrt/1
  y/1 -> Square/1
  Square/1 -> Sum/1
  Square1/1 -> Sum/2
  Sqrt/1 -> Crosstrack error/1

== system SpaceRendezvousAndDockingExample/Chaser spacecraft/Guidance and control/Guidance/Maneuver/Docking/Docking phase guidance/Initial approach/Translational guidance/Crosstrack error ==
  y : Inport
  z : Inport  Port=2
  Sqrt : Sqrt
  Square : Math  Operator=square
  Square1 : Math  Operator=square
  Sum : Sum
  Crosstrack error : Outport
  wires:
  z/1 -> Square1/1
  Sum/1 -> Sqrt/1
  y/1 -> Square/1
  Square/1 -> Sum/1
  Square1/1 -> Sum/2
  Sqrt/1 -> Crosstrack error/1

== system SpaceRendezvousAndDockingExample/Chaser spacecraft/Guidance and control/Guidance/Maneuver/Docking/Docking phase guidance/Transposition/Translational guidance/Norm ==
  Vector : Inport
  Dot Product : DotProduct  OutDataTypeStr=Inherit: Inherit via internal rule
  Sqrt : Sqrt
  Norm : Outport
  wires:
  Vector/1 -> Dot Product/2, Dot Product/1
  Dot Product/1 -> Sqrt/1
  Sqrt/1 -> Norm/1

== stateflow chart SpaceRendezvousAndDockingExample/Chaser spacecraft/Guidance and control/Guidance/Maneuver/Docking/Docking phase selector/Docking phase selector ==
  state InitialApproach
    entry:
    enableInitialApproach = 1;
    enableTransposition = 0;
    enableFinalApproach = 0;
    exit:
    enableInitialApproach = 0;
  state Transposition
    entry:
    enableTransposition = 1;
    exit:
    enableTransposition = 0;
  state FinalApproach
    entry:
    enableFinalApproach = 1;
  (default) -> InitialApproach
  InitialApproach -> Transposition : [relativeDistance < 100]
  Transposition -> FinalApproach : [transpositionError < 0.1]
  data: enableInitialApproach output; relativeDistance input; enableTransposition output; transpositionError input; enableFinalApproach output

== stateflow chart SpaceRendezvousAndDockingExample/Chaser spacecraft/Guidance and control/Guidance/Maneuver selector ==
  state Maneuver1
    entry:
    enableRendezvousManeuver1 = 1;
    enableRendezvousManeuver2 = 0;
    enableDocking = 0;
    exit:
    enableRendezvousManeuver1 = 0;
  state Maneuver2
    entry:
    enableRendezvousManeuver2 = 1;
    exit:
    enableRendezvousManeuver2 = 0;
  state RendezvousAndDocking
    entry:
    enableDocking = 1;
  (default) -> Maneuver1
  Maneuver1 -> Maneuver2 : [missionTime>(burnTime1+burnDuration1)]
  Maneuver2 -> RendezvousAndDocking : [missionTime>(burnTime2+burnDuration2)]
  data: enableRendezvousManeuver1 output; enableRendezvousManeuver2 output; burnDuration1 parameter; burnDuration2 parameter; burnTime2 parameter; burnTime1 parameter; missionTime input; enableDocking output
